simulink model "GEMV_Stream_Ex5"  (R2026a)
settings: Solver=VariableStepAuto  StopTime=10
undefined symbols (not defined in the file): Column, L, major, vsva1596, xcvc1702
libraries: aieDSP x1, aieUtilities x1, vmcUtilities x1
settings Model: Creator=sdegala  LastModifiedBy=robg

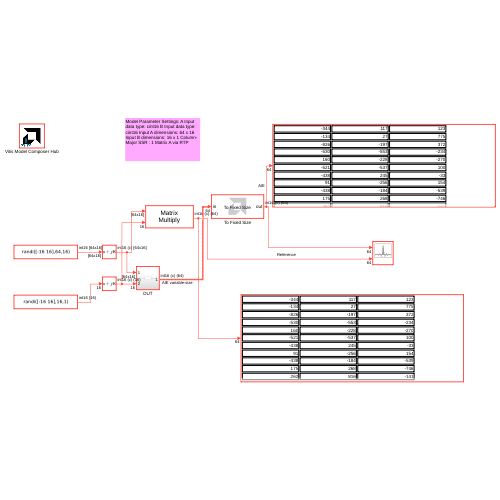
[thumbnail: Simulink's stored preview of the top-level diagram]
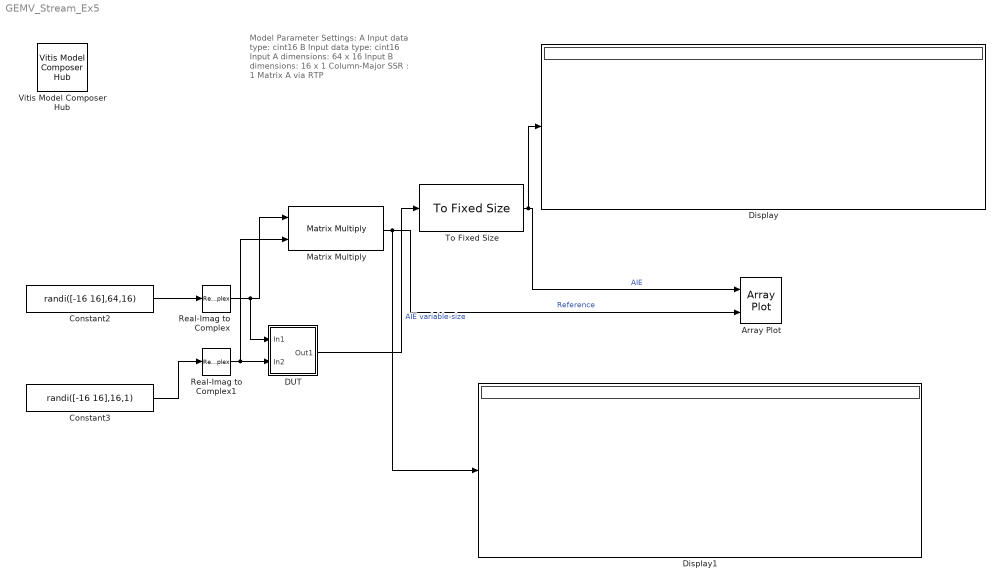
== system GEMV_Stream_Ex5 ==
  note: Model Parameter Settings:
      |
      | A Input data type: cint16
      | B Input data type: cint16
      | Input A dimensions: 64 x 16
      | Input B dimensions: 16 x 1
      | Column-Major
      | SSR : 1
      | Matrix A via RTP
  Array Plot : ArrayPlot  NumInputPorts=2  WindowPosition=[560.000000,350.000000,800.000000,500.000000,]  Visible=on  ScopeFrameLocation=window  YLimits=[-1039.25 1093.25]  ShowLegend=on
  Constant2 : Constant  Value=randi([-16 16],64,16)  OutDataTypeStr=int16  SampleTime=1
  Constant3 : Constant  Value=randi([-16 16],16,1)  OutDataTypeStr=int16  SampleTime=1
  DUT : Subsystem
  Display : Display
  Display1 : Display
  Matrix Multiply : Product  Multiplication=Matrix(*)  OutDataTypeStr=int16
  Real-Imag to Complex : RealImagToComplex  Input=Real
  Real-Imag to Complex1 : RealImagToComplex  Input=Real
  To Fixed Size : aieUtilities/To Fixed Size  Mode=Stop simulation when input variable-size signal is not full  OutputSize=Inherit: Same as input  CopyMethod=Buffer samples to form output  HasStatusOutput=on
  Vitis Model Composer Hub : vmcUtilities/Vitis Model Composer Hub  Tag=genX  CodeGeneration=off  SubsystemName=DUT  BlockHierPath=GEMV_Stream_Ex5/DUT  SubsystemType=AIENode  StartColumn=1  NumberOfColumns=1  TargetDirectory=./code  exportDesign=off  analyzeDesign=on  validateDesignOnHw=off  ExportType=AI Engines  IpVendor=xilinx.com  IpLibrary=hls  IpVersion=1.0  IpHWLanguage=Verilog  AieCompilerOptions={}  AieSimulatorOptions={}  CreateTestbench=on  TestbenchStackSize=10  RunRtlSim=off  RunCSim=off  RunAieSim=off  enableSimulationTimeout=on  enableGraphIterations=on  AieSimTimeout=50000  AieGraphIterations=-1  RunAieSimProfiling=off  LaunchVitisAnalyzer=off  PlotOutput=off  RunX86Sim=off  X86SimTimeout=10  GenHwImage=off  GenLibadfXo=off  GenHwValidationCode=off  PlatformType=Not Specified  HwSystemType=Baremetal  HwValidationTarget=hw  ProjDevice=xcvc1702-vsva1596-2LP-e-L  ProjDevicePart=xcvc1702-vsva1596-2LP-e-L  AIEType=AIE  SamplePeriod=-1  ClockFrequency=200  DataPathParallelism=1  xilinxfamily=versalaicore  part=xcvc1702  speed=-2LP-e-L  package=vsva1596  directory=./netlist  testbench=off  incr_netlist=off  synthesis_tool=Vivado  clock_wrapper=Clock Enables  dbl_ovrd=According to Block Masks  dcm_input_clock_period=10  sysclk_period=10  simulink_period=1  eval_field=0  IPInfoJsonString="{\"DUTSubsystemName\":\"DUT\",\"AIESubsystem\":{\"SubsystemName\":\"DUT\",\"TargetDirectory\":\"./code\",\"AIEArrayConfig\":\"Use entire AIE array\",\"StartColumn\":\"0\",\"NumberOfColumns\":\"1\"},\"SubsystemTag\":\"AIENode\"}"  LogFileName=/proj/xhdhdstaff5/sdegala/Head1/HEAD/2026_1_Work/code/model_composer.log  NThreads=4  IPConfigFile=/tmp/vmctmp-16505700046410390857/GEMV_Ex1_Stream_ipconfig.json
  wires:
  Matrix Multiply/1 -> Array Plot/2, Display1/1  "Reference"
  DUT/1(Out1) -> To Fixed Size/1  "AIE variable-size"
  To Fixed Size/1 -> Display/1, Array Plot/1  "AIE"
  Constant2/1 -> Real-Imag to Complex/1
  Constant3/1 -> Real-Imag to Complex1/1
  Real-Imag to Complex/1 -> Matrix Multiply/1, DUT/1(In1)
  Real-Imag to Complex1/1 -> DUT/2(In2), Matrix Multiply/2

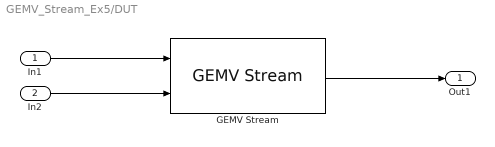
== system GEMV_Stream_Ex5/DUT ==
  In1 : Inport
  In2 : Inport  Port=2
  GEMV Stream : aieDSP/GEMV Stream  AIE_VARIANT=1  data_type_A=cint16  data_type_B=cint16  Matrix_reload=on  api=1  Dim_A=64  Dim_B=16  num_frames=1  ssr=1  casc_length=1  dual_ip=off  num_outputs=off  A_Leading_data=Column-major(1)  shift_output=0  rnd_mode=Floor  sat_mode=None  blockJsonConstraints=[]  blockJsonConstraintsInternal=[]  spec=vmc_stream_matrix_vector_mul.json  SerializedMaskParamNames=[]  SerializedMaskParamValues=[]  SerializedMaskParamVisibilities=[]  block_type=GEMV Stream  SerializedMaskParamDataypes=uint|typename|typename|uint|uint|uint|uint|uint|uint|uint|uint|uint|uint|uint|uint|uint  SerializedMaskParamEnumStrArr=0|0|0|0|0|0|0|0|0|0|0|0|Row-major(0),Column-major(1)|0|Floor,Ceiling,Round to positive infinity,Round to negative infinity,Round symmetrical to infinity,Round symmetrical to zero,Round convergent to even,Round convergent to odd|None,Saturate,Symmetric  SerializedMaskParamEnumValArr=0|0|0|0|0|0|0|0|0|0|0|0|0,1|0|0,1,2,3,4,5,6,7|0,1,3  SerializedMaskParamVectorArr=0|0|0|0|0|0|0|0|0|0|0|0|0|0|0|0  SerializedMaskParamKeys=AIE_VARIANT|TT_DATA_A|TT_DATA_B|TP_USE_MATRIX_RELOAD|TP_API|TP_DIM_A|TP_DIM_B|TP_NUM_FRAMES|TP_SSR|TP_CASC_LEN|TP_DUAL_IP|TP_NUM_OUTPUTS|TP_DIM_A_LEADING|TP_SHIFT|TP_RND|TP_SAT
  Out1 : Outport
  wires:
  In2/1 -> GEMV Stream/2
  In1/1 -> GEMV Stream/1
  GEMV Stream/1 -> Out1/1
